simulink model "Controller_Simulation"  (R2022b)
settings: Solver=ode4  StartTime=0.0  StopTime=40  FixedStep=0.01  RelTol=1e-3
settings Model: Creator=Sahil Gaurkar  LastModifiedBy=Sahil Gaurkar

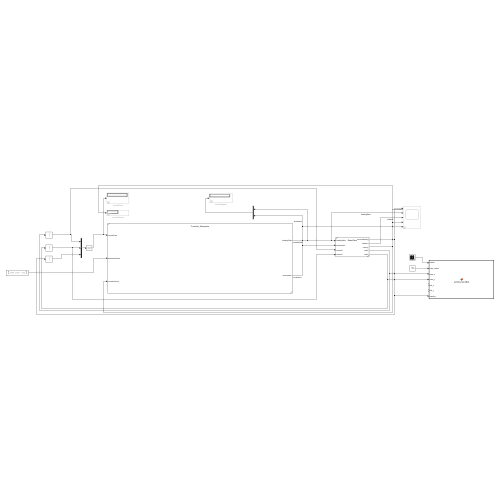
[thumbnail: Simulink's stored preview of the top-level diagram]
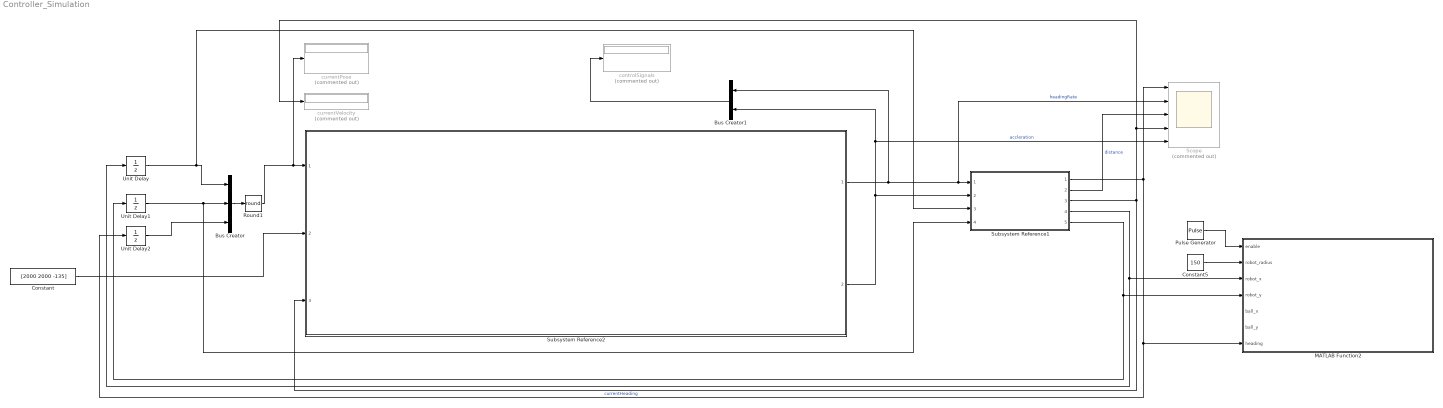
== system Controller_Simulation ==
  Bus Creator : BusCreator  Inputs=3
  Bus Creator1 : BusCreator  Inputs=2
  Constant : Constant  Value=[2000 2000 -135]
  Constant5 : Constant  Value=150
  MATLAB Function2 : MATLAB Function  InitFcn=|  TreatAsAtomicUnit=on
      | figure(1); 
      | clf;
      | hold on; 
      | grid on; 
      | axis([-45,45,-30,30]);
  Pulse Generator : DiscretePulseGenerator  PulseType=Time based  Period=1
  Round1 : Rounding  Operator=round
  Scope : Scope  Commented=on  NumInputPorts=5
  Subsystem Reference1 : Subsystem  ReferencedSubsystem=RobotPlant
  Subsystem Reference2 : Subsystem  ReferencedSubsystem=Controller_Subsystem
  Unit Delay : UnitDelay  InitialCondition=2433  SampleTime=-1  HasFrameUpgradeWarning=on
  Unit Delay1 : UnitDelay  InitialCondition=-1234  SampleTime=-1  HasFrameUpgradeWarning=on
  Unit Delay2 : UnitDelay  InitialCondition=179  SampleTime=-1  HasFrameUpgradeWarning=on
  controlSignals : Display  Commented=on
  currentPose : Display  Commented=on
  currentVelocity : Display  Commented=on
  wires:
  Unit Delay2/1 -> Bus Creator/3
  Constant/1 -> Subsystem Reference2/2
  Unit Delay1/1 -> Subsystem Reference1/4, Bus Creator/2
  Subsystem Reference2/2 -> Bus Creator1/2, Scope/5, Subsystem Reference1/2  "accleration"
  Bus Creator1/1 -> controlSignals/1
  Bus Creator/1 -> Round1/1
  Subsystem Reference2/1 -> Scope/2, Subsystem Reference1/1, Bus Creator1/1  "headingRate"
  Subsystem Reference1/1 -> MATLAB Function2/7(heading), Unit Delay2/1, Scope/1  "currentHeading"
  Subsystem Reference1/2 -> Scope/3  "distance"
  Subsystem Reference1/3 -> Subsystem Reference2/3, Scope/4, currentVelocity/1
  Subsystem Reference1/5 -> MATLAB Function2/4(robot_y), Unit Delay1/1
  Constant5/1 -> MATLAB Function2/2(robot_radius)
  Subsystem Reference1/4 -> MATLAB Function2/3(robot_x), Unit Delay/1
  Unit Delay/1 -> Bus Creator/1, Subsystem Reference1/3
  Round1/1 -> currentPose/1, Subsystem Reference2/1
  Pulse Generator/1 -> MATLAB Function2/1(enable)

== matlab function Controller_Simulation/MATLAB Function2 ==
  data: enable input; robot_radius input; robot_x input; robot_y input; ball_x input; ball_y input; heading input
function plotRobotAndBall(enable, robot_radius, robot_x, robot_y, ball_x, ball_y, heading)

if enable == 1
    figure(1);
    clf;
    hold on;
    grid on;
    axis([-9000,9000,-3000,3000]);

    theta = linspace(0, 2*pi, 360);
    heading_line_length = 300; % L

    % equation of circle for representing robot
    robot_rep_x = robot_radius * cos(theta);
    robot_rep_y = robot_radius * sin(theta);

    heading_line_x = cos((heading*pi)/180) * heading_line_length;
    heading_line_y = sin((heading*pi)/180) * heading_line_length;

    % Draw circle around current location of robot
    plot((robot_rep_x + robot_x), (robot_rep_y + robot_y), 'Color', 'b');

    % Draw line from center of robot in the direction of the current heading
    line([robot_x,  robot_x + heading_line_x], [robot_y, robot_y + heading_line_y], 'color', 'b');

    % Plot ball
    plot(ball_x, ball_y,'Color','r','Marker','o')

    drawnow();

end


end
